simulink model "LinearizedModel"  (R2025a)
settings: Solver=ode4  StartTime=0.0  StopTime=100  RelTol=1e-3
values from neighbouring files (symbols this model uses):
  Ac = [0,0,1,0 ... (first row only)    [init_linearization.m]
  Bc = [0,0 ... (first row only)    [init_linearization.m]
  psi_op = pi/2    (= 1.57079632679)    [init_linearization.m]
  theta_op = -10*pi/180    (= -0.174532925199)    [init_linearization.m]
settings Model: Creator=bulve  LastModifiedBy=BjørnErikUlveraker

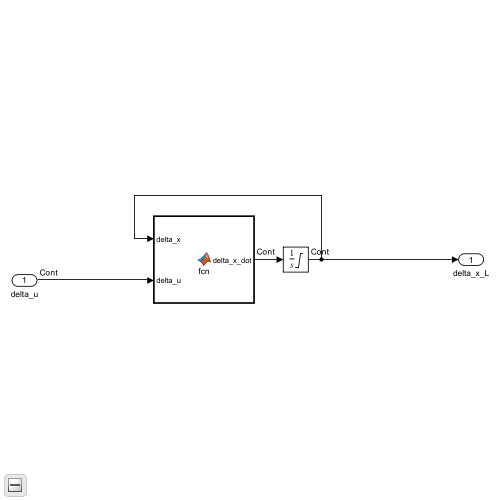
[thumbnail: Simulink's stored preview of the top-level diagram]
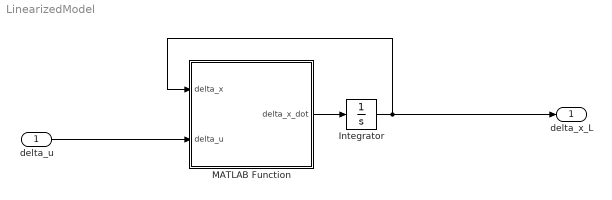
== system LinearizedModel ==
  delta_u : Inport
  Integrator : Integrator  LimitOutput=on  UpperSaturationLimit=[45*pi/180-theta_op;pi-psi_op;inf;inf]  LowerSaturationLimit=[-45*pi/180-theta_op;0-psi_op;-inf;-inf]
  MATLAB Function : MATLAB Function  TreatAsAtomicUnit=on
  delta_x_L : Outport
  wires:
  delta_u/1 -> MATLAB Function/2(delta_u)
  Integrator/1 -> MATLAB Function/1(delta_x), delta_x_L/1
  MATLAB Function/1(delta_x_dot) -> Integrator/1

== matlab function LinearizedModel/MATLAB Function ==
  data: delta_x input size=[4 1]; delta_x_dot output size=[4 1]; delta_u input size=[2 1]; Ac parameter; Bc parameter

function delta_x_dot = fcn(delta_x, delta_u, Ac, Bc)

delta_x_dot = Ac*delta_x + Bc*delta_u;
